simulink model "simulazione_punto_4"  (R2025b)
settings: Solver=VariableStepAuto  StartTime=0.0  StopTime=10.0  RelTol=1e-3
values from neighbouring files (symbols this model uses):
  G = tf(modello)    [tank_in_cascata_costanti.m]
  RR = RR_s*RR_d    [tank_in_cascata_costanti.m]
settings Model: Creator=lucia  LastModifiedBy=lucia

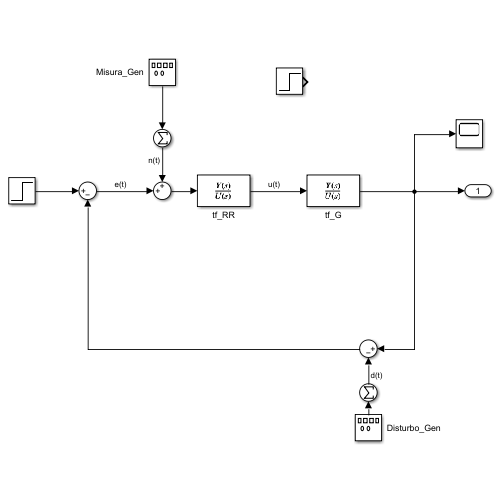
[thumbnail: Simulink's stored preview of the top-level diagram]
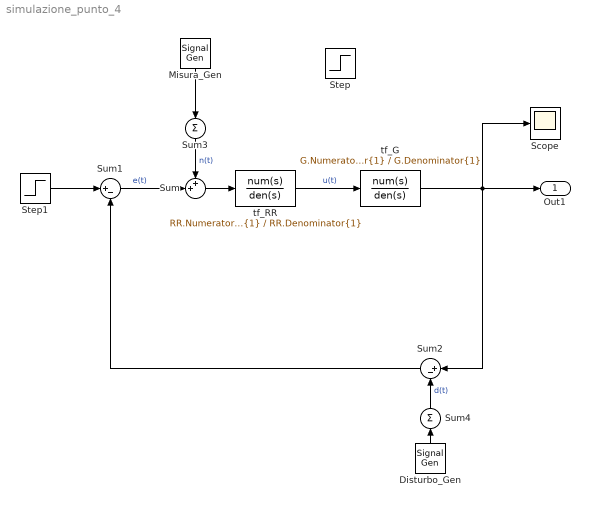
== system simulazione_punto_4 ==
  Disturbo_Gen : SignalGenerator  Amplitude=1.5  Frequency="[0.4         0.8         1.2         1.6]"  Units=rad/sec
  Misura_Gen : SignalGenerator  Amplitude=0.1  Frequency="[200000  400000  600000  800000]"  Units=rad/sec
  Scope : Scope
  Step : Step  SampleTime=0
  Step1 : Step  SampleTime=0
  Sum : Sum  Inputs=++|
  Sum1 : Sum  Inputs=|+-
  Sum2 : Sum  Inputs=|+-
  Sum3 : Sum  Inputs=+
  Sum4 : Sum  Inputs=+
  tf_G : TransferFcn  Numerator=G.Numerator{1}  Denominator=G.Denominator{1}
  tf_RR : TransferFcn  Numerator=RR.Numerator{1}  Denominator=RR.Denominator{1}
  Out1 : Outport
  wires:
  tf_RR/1 -> tf_G/1  "u(t)"
  tf_G/1 -> Scope/1, Sum2/1, Out1/1
  Sum1/1 -> Sum/2  "e(t)"
  Sum/1 -> tf_RR/1
  Misura_Gen/1 -> Sum3/1
  Sum3/1 -> Sum/1  "n(t)"
  Disturbo_Gen/1 -> Sum4/1
  Sum4/1 -> Sum2/2  "d(t)"
  Sum2/1 -> Sum1/2
  Step1/1 -> Sum1/1
